simulink model "MdXX_RspOutComm"  (R2022b)
settings: Solver=FixedStepDiscrete  StartTime=0.0  StopTime=10.0  FixedStep=0.01  RelTol=1e-3
undefined symbols (not defined in the file or in its folder): KeSMSuRspStatHldTm_Val, MdRspLocal2, SrcReqTp1
libraries: simulink x64, RspLib x32
(part 2 of 5)

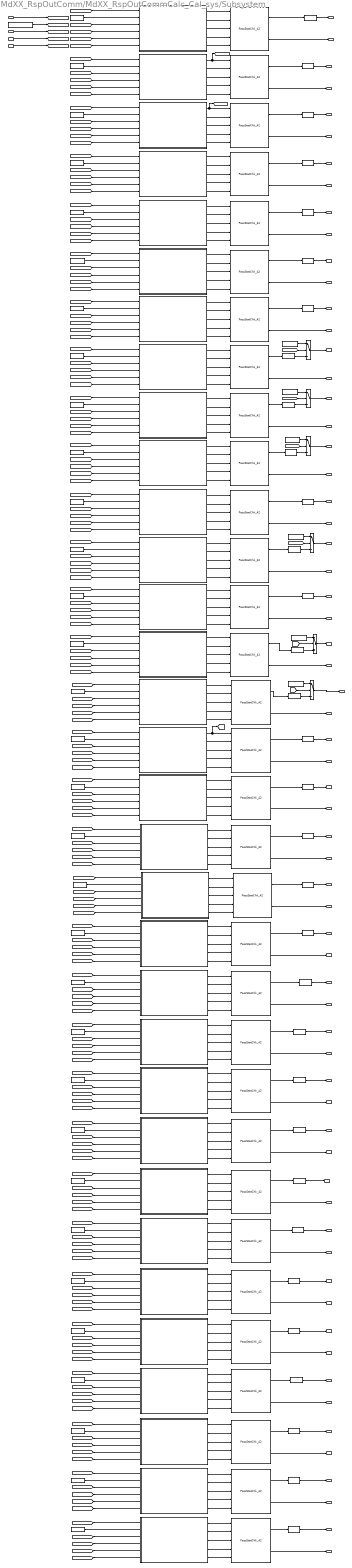
== system MdXX_RspOutComm/MdXX_RspOutCommCalc_Cal_sys/Subsystem ==
  MdXXIsTargetPosAlready_Val_read : Inport
  modestate32_Val_read : Inport  Port=2
  MdXX_QuitArray_Val_read : Inport  Port=3
  MdXX_SrcReqTpArray_Val_read : Inport  Port=4
  Constant{,32..37} (7 alike) : Constant  Value=0  OutDataTypeStr=uint8
  Constant1 : Constant  OutDataTypeStr=uint8
  Constant10 : Constant  Value=10  OutDataTypeStr=uint8
  Constant11 : Constant  Value=11  OutDataTypeStr=uint8
  Constant12 : Constant  Value=12  OutDataTypeStr=uint8
  Constant13 : Constant  Value=13  OutDataTypeStr=uint8
  Constant14 : Constant  Value=14  OutDataTypeStr=uint8
  Constant15 : Constant  Value=15  OutDataTypeStr=uint8
  Constant16 : Constant  Value=16  OutDataTypeStr=uint8
  Constant17 : Constant  Value=17  OutDataTypeStr=uint8
  Constant18 : Constant  Value=18  OutDataTypeStr=uint8
  Constant19 : Constant  Value=19  OutDataTypeStr=uint8
  Constant2 : Constant  Value=2  OutDataTypeStr=uint8
  Constant20 : Constant  Value=20  OutDataTypeStr=uint8
  Constant21 : Constant  Value=21  OutDataTypeStr=uint8
  Constant22 : Constant  Value=22  OutDataTypeStr=uint8
  Constant23 : Constant  Value=23  OutDataTypeStr=uint8
  Constant24 : Constant  Value=24  OutDataTypeStr=uint8
  Constant25 : Constant  Value=25  OutDataTypeStr=uint8
  Constant26 : Constant  Value=26  OutDataTypeStr=uint8
  Constant27 : Constant  Value=27  OutDataTypeStr=uint8
  Constant28 : Constant  Value=28  OutDataTypeStr=uint8
  Constant29 : Constant  Value=29  OutDataTypeStr=uint8
  Constant3 : Constant  Value=3  OutDataTypeStr=uint8
  Constant30 : Constant  Value=30  OutDataTypeStr=uint8
  Constant31 : Constant  Value=31  OutDataTypeStr=uint8
  Constant4 : Constant  Value=4  OutDataTypeStr=uint8
  Constant5 : Constant  Value=5  OutDataTypeStr=uint8
  Constant6 : Constant  Value=6  OutDataTypeStr=uint8
  Constant7 : Constant  Value=7  OutDataTypeStr=uint8
  Constant8 : Constant  Value=8  OutDataTypeStr=uint8
  Constant9 : Constant  Value=9  OutDataTypeStr=uint8
  Data Type Conversion{1..32} (32 alike) : DataTypeConversion  OutDataTypeStr=uint8  SaturateOnIntegerOverflow=off  RndMeth=Floor
  MdRsp{1..32} (32 alike) : RspLib/PassStatChk_42  SystemSampleTime=-1  VariantActivationTime=update diagram  Latency=0  AutoFrameSizeCalculation=off
  MdRspOutDataSelc1 : Subsystem
  MdRspOutDataSelc10 : Subsystem
  MdRspOutDataSelc11 : Subsystem
  MdRspOutDataSelc12 : Subsystem
  MdRspOutDataSelc13 : Subsystem
  MdRspOutDataSelc14 : Subsystem
  MdRspOutDataSelc15 : Subsystem
  MdRspOutDataSelc16 : Subsystem
  MdRspOutDataSelc17 : Subsystem
  MdRspOutDataSelc18 : Subsystem
  MdRspOutDataSelc19 : Subsystem
  MdRspOutDataSelc2 : Subsystem
  MdRspOutDataSelc20 : Subsystem
  MdRspOutDataSelc21 : Subsystem
  MdRspOutDataSelc22 : Subsystem
  MdRspOutDataSelc23 : Subsystem
  MdRspOutDataSelc24 : Subsystem
  MdRspOutDataSelc25 : Subsystem
  MdRspOutDataSelc26 : Subsystem
  MdRspOutDataSelc27 : Subsystem
  MdRspOutDataSelc28 : Subsystem
  MdRspOutDataSelc29 : Subsystem
  MdRspOutDataSelc3 : Subsystem
  MdRspOutDataSelc30 : Subsystem
  MdRspOutDataSelc31 : Subsystem
  MdRspOutDataSelc32 : Subsystem
  MdRspOutDataSelc4 : Subsystem
  MdRspOutDataSelc5 : Subsystem
  MdRspOutDataSelc6 : Subsystem
  MdRspOutDataSelc7 : Subsystem
  MdRspOutDataSelc8 : Subsystem
  MdRspOutDataSelc9 : Subsystem
  PA_KeSMSuRspStatHldTm_Val : Constant  Value=KeSMSuRspStatHldTm_Val
  Switch{,1..5} (6 alike) : Switch  Criteria=u2 > Threshold  SaturateOnIntegerOverflow=off  InputSameDT=off
  MdXX_RspOutComm_Md1_Rsp_write : Outport  VectorParamsAs1DForOutWhenUnconnected=off
      settings: EnsureOutportIsVirtual=on
  MdXX_RspOutComm_Md10_Rsp_write : Outport  Port=2  VectorParamsAs1DForOutWhenUnconnected=off
      settings: EnsureOutportIsVirtual=on
  MdXX_RspOutComm_Md11_Rsp_write : Outport  Port=3  VectorParamsAs1DForOutWhenUnconnected=off
      settings: EnsureOutportIsVirtual=on
  MdXX_RspOutComm_Md12_Rsp_write : Outport  Port=4  VectorParamsAs1DForOutWhenUnconnected=off
      settings: EnsureOutportIsVirtual=on
  MdXX_RspOutComm_Md13_Rsp_write : Outport  Port=5  VectorParamsAs1DForOutWhenUnconnected=off
      settings: EnsureOutportIsVirtual=on
  MdXX_RspOutComm_Md14_Rsp_write : Outport  Port=6  VectorParamsAs1DForOutWhenUnconnected=off
      settings: EnsureOutportIsVirtual=on
  MdXX_RspOutComm_Md15_Rsp_write : Outport  Port=7  VectorParamsAs1DForOutWhenUnconnected=off
      settings: EnsureOutportIsVirtual=on
  MdXX_RspOutComm_Md16_Rsp_write : Outport  Port=8  VectorParamsAs1DForOutWhenUnconnected=off
      settings: EnsureOutportIsVirtual=on
  MdXX_RspOutComm_Md17_Rsp_write : Outport  Port=9  VectorParamsAs1DForOutWhenUnconnected=off
      settings: EnsureOutportIsVirtual=on
  MdXX_RspOutComm_Md18_Rsp_write : Outport  Port=10  VectorParamsAs1DForOutWhenUnconnected=off
      settings: EnsureOutportIsVirtual=on
  MdXX_RspOutComm_Md19_Rsp_write : Outport  Port=11  VectorParamsAs1DForOutWhenUnconnected=off
      settings: EnsureOutportIsVirtual=on
  MdXX_RspOutComm_Md2_Rsp_write : Outport  Port=12  VectorParamsAs1DForOutWhenUnconnected=off
      settings: EnsureOutportIsVirtual=on
  MdXX_RspOutComm_Md20_Rsp_write : Outport  Port=13  VectorParamsAs1DForOutWhenUnconnected=off
      settings: EnsureOutportIsVirtual=on
  MdXX_RspOutComm_Md21_Rsp_write : Outport  Port=14  VectorParamsAs1DForOutWhenUnconnected=off
      settings: EnsureOutportIsVirtual=on
  MdXX_RspOutComm_Md22_Rsp_write : Outport  Port=15  VectorParamsAs1DForOutWhenUnconnected=off
      settings: EnsureOutportIsVirtual=on
  MdXX_RspOutComm_Md23_Rsp_write : Outport  Port=16  VectorParamsAs1DForOutWhenUnconnected=off
      settings: EnsureOutportIsVirtual=on
  MdXX_RspOutComm_Md24_Rsp_write : Outport  Port=17  VectorParamsAs1DForOutWhenUnconnected=off
      settings: EnsureOutportIsVirtual=on
  MdXX_RspOutComm_Md25_Rsp_write : Outport  Port=18  VectorParamsAs1DForOutWhenUnconnected=off
      settings: EnsureOutportIsVirtual=on
  MdXX_RspOutComm_Md26_Rsp_write : Outport  Port=19  VectorParamsAs1DForOutWhenUnconnected=off
      settings: EnsureOutportIsVirtual=on
  MdXX_RspOutComm_Md27_Rsp_write : Outport  Port=20  VectorParamsAs1DForOutWhenUnconnected=off
      settings: EnsureOutportIsVirtual=on
  MdXX_RspOutComm_Md28_Rsp_write : Outport  Port=21  VectorParamsAs1DForOutWhenUnconnected=off
      settings: EnsureOutportIsVirtual=on
  MdXX_RspOutComm_Md29_Rsp_write : Outport  Port=22  VectorParamsAs1DForOutWhenUnconnected=off
      settings: EnsureOutportIsVirtual=on
  MdXX_RspOutComm_Md3_Rsp_write : Outport  Port=23  VectorParamsAs1DForOutWhenUnconnected=off
      settings: EnsureOutportIsVirtual=on
  MdXX_RspOutComm_Md30_Rsp_write : Outport  Port=24  VectorParamsAs1DForOutWhenUnconnected=off
      settings: EnsureOutportIsVirtual=on
  MdXX_RspOutComm_Md31_Rsp_write : Outport  Port=25  VectorParamsAs1DForOutWhenUnconnected=off
      settings: EnsureOutportIsVirtual=on
  MdXX_RspOutComm_Md32_Rsp_write : Outport  Port=26  VectorParamsAs1DForOutWhenUnconnected=off
      settings: EnsureOutportIsVirtual=on
  MdXX_RspOutComm_Md4_Rsp_write : Outport  Port=27  VectorParamsAs1DForOutWhenUnconnected=off
      settings: EnsureOutportIsVirtual=on
  MdXX_RspOutComm_Md5_Rsp_write : Outport  Port=28  VectorParamsAs1DForOutWhenUnconnected=off
      settings: EnsureOutportIsVirtual=on
  MdXX_RspOutComm_Md6_Rsp_write : Outport  Port=29  VectorParamsAs1DForOutWhenUnconnected=off
      settings: EnsureOutportIsVirtual=on
  MdXX_RspOutComm_Md7_Rsp_write : Outport  Port=30  VectorParamsAs1DForOutWhenUnconnected=off
      settings: EnsureOutportIsVirtual=on
  MdXX_RspOutComm_Md8_Rsp_write : Outport  Port=31  VectorParamsAs1DForOutWhenUnconnected=off
      settings: EnsureOutportIsVirtual=on
  MdXX_RspOutComm_Md9_Rsp_write : Outport  Port=32  VectorParamsAs1DForOutWhenUnconnected=off
      settings: EnsureOutportIsVirtual=on
  MdXX_SrcReqTpOutComm_Md1_SrcTp_write : Outport  Port=33  VectorParamsAs1DForOutWhenUnconnected=off
      settings: EnsureOutportIsVirtual=on
  MdXX_SrcReqTpOutComm_Md10_SrcTp_write : Outport  Port=34  VectorParamsAs1DForOutWhenUnconnected=off
      settings: EnsureOutportIsVirtual=on
  MdXX_SrcReqTpOutComm_Md11_SrcTp_write : Outport  Port=35  VectorParamsAs1DForOutWhenUnconnected=off
      settings: EnsureOutportIsVirtual=on
  MdXX_SrcReqTpOutComm_Md12_SrcTp_write : Outport  Port=36  VectorParamsAs1DForOutWhenUnconnected=off
      settings: EnsureOutportIsVirtual=on
  MdXX_SrcReqTpOutComm_Md13_SrcTp_write : Outport  Port=37  VectorParamsAs1DForOutWhenUnconnected=off
      settings: EnsureOutportIsVirtual=on
  MdXX_SrcReqTpOutComm_Md14_SrcTp_write : Outport  Port=38  VectorParamsAs1DForOutWhenUnconnected=off
      settings: EnsureOutportIsVirtual=on
  MdXX_SrcReqTpOutComm_Md15_SrcTp_write : Outport  Port=39  VectorParamsAs1DForOutWhenUnconnected=off
      settings: EnsureOutportIsVirtual=on
  MdXX_SrcReqTpOutComm_Md16_SrcTp_write : Outport  Port=40  VectorParamsAs1DForOutWhenUnconnected=off
      settings: EnsureOutportIsVirtual=on
  MdXX_SrcReqTpOutComm_Md17_SrcTp_write : Outport  Port=41  VectorParamsAs1DForOutWhenUnconnected=off
      settings: EnsureOutportIsVirtual=on
  MdXX_SrcReqTpOutComm_Md18_SrcTp_write : Outport  Port=42  VectorParamsAs1DForOutWhenUnconnected=off
      settings: EnsureOutportIsVirtual=on
  MdXX_SrcReqTpOutComm_Md19_SrcTp_write : Outport  Port=43  VectorParamsAs1DForOutWhenUnconnected=off
      settings: EnsureOutportIsVirtual=on
  MdXX_SrcReqTpOutComm_Md2_SrcTp_write : Outport  Port=44  VectorParamsAs1DForOutWhenUnconnected=off
      settings: EnsureOutportIsVirtual=on
  MdXX_SrcReqTpOutComm_Md20_SrcTp_write : Outport  Port=45  VectorParamsAs1DForOutWhenUnconnected=off
      settings: EnsureOutportIsVirtual=on
  MdXX_SrcReqTpOutComm_Md21_SrcTp_write : Outport  Port=46  VectorParamsAs1DForOutWhenUnconnected=off
      settings: EnsureOutportIsVirtual=on
  MdXX_SrcReqTpOutComm_Md22_SrcTp_write : Outport  Port=47  VectorParamsAs1DForOutWhenUnconnected=off
      settings: EnsureOutportIsVirtual=on
  MdXX_SrcReqTpOutComm_Md23_SrcTp_write : Outport  Port=48  VectorParamsAs1DForOutWhenUnconnected=off
      settings: EnsureOutportIsVirtual=on
  MdXX_SrcReqTpOutComm_Md24_SrcTp_write : Outport  Port=49  VectorParamsAs1DForOutWhenUnconnected=off
      settings: EnsureOutportIsVirtual=on
  MdXX_SrcReqTpOutComm_Md25_SrcTp_write : Outport  Port=50  VectorParamsAs1DForOutWhenUnconnected=off
      settings: EnsureOutportIsVirtual=on
  MdXX_SrcReqTpOutComm_Md26_SrcTp_write : Outport  Port=51  VectorParamsAs1DForOutWhenUnconnected=off
      settings: EnsureOutportIsVirtual=on
  MdXX_SrcReqTpOutComm_Md27_SrcTp_write : Outport  Port=52  VectorParamsAs1DForOutWhenUnconnected=off
      settings: EnsureOutportIsVirtual=on
  MdXX_SrcReqTpOutComm_Md28_SrcTp_write : Outport  Port=53  VectorParamsAs1DForOutWhenUnconnected=off
      settings: EnsureOutportIsVirtual=on
  MdXX_SrcReqTpOutComm_Md29_SrcTp_write : Outport  Port=54  VectorParamsAs1DForOutWhenUnconnected=off
      settings: EnsureOutportIsVirtual=on
  MdXX_SrcReqTpOutComm_Md3_SrcTp_write : Outport  Port=55  VectorParamsAs1DForOutWhenUnconnected=off
      settings: EnsureOutportIsVirtual=on
  MdXX_SrcReqTpOutComm_Md30_SrcTp_write : Outport  Port=56  VectorParamsAs1DForOutWhenUnconnected=off
      settings: EnsureOutportIsVirtual=on
  MdXX_SrcReqTpOutComm_Md31_SrcTp_write : Outport  Port=57  VectorParamsAs1DForOutWhenUnconnected=off
      settings: EnsureOutportIsVirtual=on
  MdXX_SrcReqTpOutComm_Md32_SrcTp_write : Outport  Port=58  VectorParamsAs1DForOutWhenUnconnected=off
      settings: EnsureOutportIsVirtual=on
  MdXX_SrcReqTpOutComm_Md4_SrcTp_write : Outport  Port=59  VectorParamsAs1DForOutWhenUnconnected=off
      settings: EnsureOutportIsVirtual=on
  MdXX_SrcReqTpOutComm_Md5_SrcTp_write : Outport  Port=60  VectorParamsAs1DForOutWhenUnconnected=off
      settings: EnsureOutportIsVirtual=on
  MdXX_SrcReqTpOutComm_Md6_SrcTp_write : Outport  Port=61  VectorParamsAs1DForOutWhenUnconnected=off
      settings: EnsureOutportIsVirtual=on
  MdXX_SrcReqTpOutComm_Md7_SrcTp_write : Outport  Port=62  VectorParamsAs1DForOutWhenUnconnected=off
      settings: EnsureOutportIsVirtual=on
  MdXX_SrcReqTpOutComm_Md8_SrcTp_write : Outport  Port=63  VectorParamsAs1DForOutWhenUnconnected=off
      settings: EnsureOutportIsVirtual=on
  MdXX_SrcReqTpOutComm_Md9_SrcTp_write : Outport  Port=64  VectorParamsAs1DForOutWhenUnconnected=off
      settings: EnsureOutportIsVirtual=on
  wires:
  MdRsp16/1 -> Data Type Conversion16/1
  MdRsp10/1 -> Data Type Conversion10/1
  MdRsp13/1 -> Data Type Conversion13/1
  MdRsp18/1 -> Data Type Conversion18/1
  MdRsp12/1 -> Data Type Conversion12/1
  MdRsp17/1 -> Data Type Conversion17/1
  MdRsp19/1 -> Data Type Conversion19/1
  MdRsp11/1 -> Data Type Conversion11/1
  MdRsp20/1 -> Data Type Conversion20/1
  MdRsp1/1 -> Data Type Conversion1/1
  MdRsp2/1 -> Data Type Conversion2/1
  MdRsp3/1 -> Data Type Conversion4/1
  MdRsp4/1 -> Data Type Conversion3/1
  MdRsp5/1 -> Data Type Conversion5/1
  MdRsp6/1 -> Data Type Conversion6/1
  MdRsp7/1 -> Data Type Conversion7/1
  MdRsp8/1 -> Data Type Conversion8/1
  MdRsp9/1 -> Data Type Conversion9/1
  MdRsp1/2 -> MdXX_SrcReqTpOutComm_Md1_SrcTp_write/1
  MdRsp4/2 -> MdXX_SrcReqTpOutComm_Md4_SrcTp_write/1
  MdRsp5/2 -> MdXX_SrcReqTpOutComm_Md5_SrcTp_write/1
  MdRsp6/2 -> MdXX_SrcReqTpOutComm_Md6_SrcTp_write/1
  MdRsp7/2 -> MdXX_SrcReqTpOutComm_Md7_SrcTp_write/1
  MdRsp8/2 -> MdXX_SrcReqTpOutComm_Md8_SrcTp_write/1
  MdRsp9/2 -> MdXX_SrcReqTpOutComm_Md9_SrcTp_write/1
  MdRsp10/2 -> MdXX_SrcReqTpOutComm_Md10_SrcTp_write/1
  MdRsp11/2 -> MdXX_SrcReqTpOutComm_Md11_SrcTp_write/1
  MdRsp12/2 -> MdXX_SrcReqTpOutComm_Md12_SrcTp_write/1
  MdRsp13/2 -> MdXX_SrcReqTpOutComm_Md13_SrcTp_write/1
  MdRsp14/2 -> MdXX_SrcReqTpOutComm_Md14_SrcTp_write/1
  MdRsp15/2 -> MdXX_SrcReqTpOutComm_Md15_SrcTp_write/1
  MdRsp16/2 -> MdXX_SrcReqTpOutComm_Md16_SrcTp_write/1
  MdRsp17/2 -> MdXX_SrcReqTpOutComm_Md17_SrcTp_write/1
  MdRsp18/2 -> MdXX_SrcReqTpOutComm_Md18_SrcTp_write/1
  MdRsp19/2 -> MdXX_SrcReqTpOutComm_Md19_SrcTp_write/1
  MdRsp20/2 -> MdXX_SrcReqTpOutComm_Md20_SrcTp_write/1
  MdRsp2/2 -> MdXX_SrcReqTpOutComm_Md2_SrcTp_write/1
  MdRsp3/2 -> MdXX_SrcReqTpOutComm_Md3_SrcTp_write/1
  Data Type Conversion3/1 -> MdXX_RspOutComm_Md4_Rsp_write/1
  Data Type Conversion4/1 -> MdXX_RspOutComm_Md3_Rsp_write/1
  Data Type Conversion2/1 -> MdXX_RspOutComm_Md2_Rsp_write/1
  Data Type Conversion1/1 -> MdXX_RspOutComm_Md1_Rsp_write/1
  Data Type Conversion5/1 -> MdXX_RspOutComm_Md5_Rsp_write/1
  Data Type Conversion6/1 -> MdXX_RspOutComm_Md6_Rsp_write/1
  Data Type Conversion7/1 -> MdXX_RspOutComm_Md7_Rsp_write/1
  Data Type Conversion11/1 -> MdXX_RspOutComm_Md11_Rsp_write/1
  Data Type Conversion13/1 -> MdXX_RspOutComm_Md13_Rsp_write/1
  Switch5/1 -> MdXX_RspOutComm_Md15_Rsp_write/1
  Data Type Conversion16/1 -> MdXX_RspOutComm_Md16_Rsp_write/1
  Data Type Conversion17/1 -> MdXX_RspOutComm_Md17_Rsp_write/1
  Data Type Conversion18/1 -> MdXX_RspOutComm_Md18_Rsp_write/1
  Data Type Conversion19/1 -> MdXX_RspOutComm_Md19_Rsp_write/1
  Data Type Conversion20/1 -> MdXX_RspOutComm_Md20_Rsp_write/1
  MdRsp32/2 -> MdXX_SrcReqTpOutComm_Md32_SrcTp_write/1
  MdRsp31/2 -> MdXX_SrcReqTpOutComm_Md31_SrcTp_write/1
  MdRsp30/2 -> MdXX_SrcReqTpOutComm_Md30_SrcTp_write/1
  MdRsp29/2 -> MdXX_SrcReqTpOutComm_Md29_SrcTp_write/1
  MdRsp28/2 -> MdXX_SrcReqTpOutComm_Md28_SrcTp_write/1
  MdRsp27/2 -> MdXX_SrcReqTpOutComm_Md27_SrcTp_write/1
  MdRsp26/2 -> MdXX_SrcReqTpOutComm_Md26_SrcTp_write/1
  MdRsp25/2 -> MdXX_SrcReqTpOutComm_Md25_SrcTp_write/1
  MdRsp24/2 -> MdXX_SrcReqTpOutComm_Md24_SrcTp_write/1
  MdRsp23/2 -> MdXX_SrcReqTpOutComm_Md23_SrcTp_write/1
  MdRsp22/2 -> MdXX_SrcReqTpOutComm_Md22_SrcTp_write/1
  MdRsp21/2 -> MdXX_SrcReqTpOutComm_Md21_SrcTp_write/1
  MdRspOutDataSelc1/1(MdEn) -> MdRsp1/1
  MdRspOutDataSelc1/2(HldTm) -> MdRsp1/2
  MdRspOutDataSelc1/3(Rsp) -> MdRsp1/3
  MdRspOutDataSelc1/4(IsTrgtPos) -> MdRsp1/4
  MdRspOutDataSelc1/5(SrcReqTp) -> MdRsp1/5
  MdRspOutDataSelc2/5(SrcReqTp) -> MdRsp2/5
  MdRspOutDataSelc2/4(IsTrgtPos) -> MdRsp2/4
  MdRspOutDataSelc2/3(Rsp) -> MdRsp2/3
  MdRspOutDataSelc3/3(Rsp) -> MdRsp3/3
  MdRspOutDataSelc3/4(IsTrgtPos) -> MdRsp3/4
  MdRspOutDataSelc3/5(SrcReqTp) -> MdRsp3/5
  MdRspOutDataSelc4/5(SrcReqTp) -> MdRsp4/5
  MdRspOutDataSelc4/4(IsTrgtPos) -> MdRsp4/4
  MdRspOutDataSelc4/3(Rsp) -> MdRsp4/3
  MdRspOutDataSelc5/3(Rsp) -> MdRsp5/3
  MdRspOutDataSelc5/4(IsTrgtPos) -> MdRsp5/4
  MdRspOutDataSelc5/5(SrcReqTp) -> MdRsp5/5
  MdRspOutDataSelc6/5(SrcReqTp) -> MdRsp6/5
  MdRspOutDataSelc6/4(IsTrgtPos) -> MdRsp6/4
  MdRspOutDataSelc6/3(Rsp) -> MdRsp6/3
  MdRspOutDataSelc7/3(Rsp) -> MdRsp7/3
  MdRspOutDataSelc7/4(IsTrgtPos) -> MdRsp7/4
  MdRspOutDataSelc7/5(SrcReqTp) -> MdRsp7/5
  MdRspOutDataSelc8/5(SrcReqTp) -> MdRsp8/5
  MdRspOutDataSelc8/4(IsTrgtPos) -> MdRsp8/4
  MdRspOutDataSelc8/3(Rsp) -> MdRsp8/3
  MdRspOutDataSelc9/3(Rsp) -> MdRsp9/3
  MdRspOutDataSelc9/4(IsTrgtPos) -> MdRsp9/4
  MdRspOutDataSelc9/5(SrcReqTp) -> MdRsp9/5
  MdRspOutDataSelc10/5(SrcReqTp) -> MdRsp10/5
  MdRspOutDataSelc10/4(IsTrgtPos) -> MdRsp10/4
  MdRspOutDataSelc10/3(Rsp) -> MdRsp10/3
  MdRspOutDataSelc11/3(Rsp) -> MdRsp11/3
  MdRspOutDataSelc11/4(IsTrgtPos) -> MdRsp11/4
  MdRspOutDataSelc11/5(SrcReqTp) -> MdRsp11/5
  MdRspOutDataSelc12/5(SrcReqTp) -> MdRsp12/5
  MdRspOutDataSelc12/4(IsTrgtPos) -> MdRsp12/4
  MdRspOutDataSelc12/3(Rsp) -> MdRsp12/3
  MdRspOutDataSelc13/3(Rsp) -> MdRsp13/3
  MdRspOutDataSelc13/4(IsTrgtPos) -> MdRsp13/4
  MdRspOutDataSelc13/5(SrcReqTp) -> MdRsp13/5
  modestate32_Val_read/1 -> [modestate32]
  Constant/1 -> MdRspOutDataSelc1/2(Index)
  [modestate32] -> MdRspOutDataSelc1/1(modestate32_Val_read)
  PA_KeSMSuRspStatHldTm_Val/1 -> [KeSMSuRspStatHldTm_Val]
  MdXX_QuitArray_Val_read/1 -> [MdXX_QuitArray]
  MdXXIsTargetPosAlready_Val_read/1 -> [MdXXIsTargetPosAlready]
  MdXX_SrcReqTpArray_Val_read/1 -> [MdXX_SrcReqTpArray]
  [KeSMSuRspStatHldTm_Val] -> MdRspOutDataSelc1/3(KeSMSuRspStatHldTm_Val)
  [MdXX_QuitArray] -> MdRspOutDataSelc1/4(QuitArray)
  [MdXXIsTargetPosAlready] -> MdRspOutDataSelc1/5(IsTargetPos32Bit_Val_read)
  [MdXX_SrcReqTpArray] -> MdRspOutDataSelc1/6(SrcReqTpArray)
  [modestate32] -> MdRspOutDataSelc2/1(modestate32_Val_read)
  [MdXX_QuitArray] -> MdRspOutDataSelc2/4(QuitArray)
  [MdXXIsTargetPosAlready] -> MdRspOutDataSelc2/5(IsTargetPos32Bit_Val_read)
  Constant1/1 -> MdRspOutDataSelc2/2(Index)
  [MdXX_SrcReqTpArray] -> MdRspOutDataSelc2/6(SrcReqTpArray)
  [KeSMSuRspStatHldTm_Val] -> MdRspOutDataSelc2/3(KeSMSuRspStatHldTm_Val)
  [modestate32] -> MdRspOutDataSelc3/1(modestate32_Val_read)
  [MdXX_QuitArray] -> MdRspOutDataSelc3/4(QuitArray)
  [MdXXIsTargetPosAlready] -> MdRspOutDataSelc3/5(IsTargetPos32Bit_Val_read)
  Constant2/1 -> MdRspOutDataSelc3/2(Index)
  [MdXX_SrcReqTpArray] -> MdRspOutDataSelc3/6(SrcReqTpArray)
  [KeSMSuRspStatHldTm_Val] -> MdRspOutDataSelc3/3(KeSMSuRspStatHldTm_Val)
  [modestate32] -> MdRspOutDataSelc4/1(modestate32_Val_read)
  [MdXX_QuitArray] -> MdRspOutDataSelc4/4(QuitArray)
  [MdXXIsTargetPosAlready] -> MdRspOutDataSelc4/5(IsTargetPos32Bit_Val_read)
  Constant3/1 -> MdRspOutDataSelc4/2(Index)
  [MdXX_SrcReqTpArray] -> MdRspOutDataSelc4/6(SrcReqTpArray)
  [KeSMSuRspStatHldTm_Val] -> MdRspOutDataSelc4/3(KeSMSuRspStatHldTm_Val)
  [modestate32] -> MdRspOutDataSelc5/1(modestate32_Val_read)
  [MdXX_QuitArray] -> MdRspOutDataSelc5/4(QuitArray)
  [MdXXIsTargetPosAlready] -> MdRspOutDataSelc5/5(IsTargetPos32Bit_Val_read)
  Constant4/1 -> MdRspOutDataSelc5/2(Index)
  [MdXX_SrcReqTpArray] -> MdRspOutDataSelc5/6(SrcReqTpArray)
  [KeSMSuRspStatHldTm_Val] -> MdRspOutDataSelc5/3(KeSMSuRspStatHldTm_Val)
  [modestate32] -> MdRspOutDataSelc6/1(modestate32_Val_read)
  [MdXX_QuitArray] -> MdRspOutDataSelc6/4(QuitArray)
  [MdXXIsTargetPosAlready] -> MdRspOutDataSelc6/5(IsTargetPos32Bit_Val_read)
  Constant5/1 -> MdRspOutDataSelc6/2(Index)
  [MdXX_SrcReqTpArray] -> MdRspOutDataSelc6/6(SrcReqTpArray)
  [KeSMSuRspStatHldTm_Val] -> MdRspOutDataSelc6/3(KeSMSuRspStatHldTm_Val)
  [modestate32] -> MdRspOutDataSelc7/1(modestate32_Val_read)
  [MdXX_QuitArray] -> MdRspOutDataSelc7/4(QuitArray)
  [MdXXIsTargetPosAlready] -> MdRspOutDataSelc7/5(IsTargetPos32Bit_Val_read)
  Constant6/1 -> MdRspOutDataSelc7/2(Index)
  [MdXX_SrcReqTpArray] -> MdRspOutDataSelc7/6(SrcReqTpArray)
  [KeSMSuRspStatHldTm_Val] -> MdRspOutDataSelc7/3(KeSMSuRspStatHldTm_Val)
  [modestate32] -> MdRspOutDataSelc8/1(modestate32_Val_read)
  [MdXX_QuitArray] -> MdRspOutDataSelc8/4(QuitArray)
  [MdXXIsTargetPosAlready] -> MdRspOutDataSelc8/5(IsTargetPos32Bit_Val_read)
  Constant7/1 -> MdRspOutDataSelc8/2(Index)
  [MdXX_SrcReqTpArray] -> MdRspOutDataSelc8/6(SrcReqTpArray)
  [KeSMSuRspStatHldTm_Val] -> MdRspOutDataSelc8/3(KeSMSuRspStatHldTm_Val)
  [modestate32] -> MdRspOutDataSelc9/1(modestate32_Val_read)
  [MdXX_QuitArray] -> MdRspOutDataSelc9/4(QuitArray)
  [MdXXIsTargetPosAlready] -> MdRspOutDataSelc9/5(IsTargetPos32Bit_Val_read)
  Constant8/1 -> MdRspOutDataSelc9/2(Index)
  [MdXX_SrcReqTpArray] -> MdRspOutDataSelc9/6(SrcReqTpArray)
  [KeSMSuRspStatHldTm_Val] -> MdRspOutDataSelc9/3(KeSMSuRspStatHldTm_Val)
  [modestate32] -> MdRspOutDataSelc10/1(modestate32_Val_read)
  [MdXX_QuitArray] -> MdRspOutDataSelc10/4(QuitArray)
  [MdXXIsTargetPosAlready] -> MdRspOutDataSelc10/5(IsTargetPos32Bit_Val_read)
  Constant9/1 -> MdRspOutDataSelc10/2(Index)
  [MdXX_SrcReqTpArray] -> MdRspOutDataSelc10/6(SrcReqTpArray)
  [KeSMSuRspStatHldTm_Val] -> MdRspOutDataSelc10/3(KeSMSuRspStatHldTm_Val)
  [modestate32] -> MdRspOutDataSelc11/1(modestate32_Val_read)
  [MdXX_QuitArray] -> MdRspOutDataSelc11/4(QuitArray)
  [MdXXIsTargetPosAlready] -> MdRspOutDataSelc11/5(IsTargetPos32Bit_Val_read)
  Constant10/1 -> MdRspOutDataSelc11/2(Index)
  [MdXX_SrcReqTpArray] -> MdRspOutDataSelc11/6(SrcReqTpArray)
  [KeSMSuRspStatHldTm_Val] -> MdRspOutDataSelc11/3(KeSMSuRspStatHldTm_Val)
  [modestate32] -> MdRspOutDataSelc12/1(modestate32_Val_read)
  [MdXX_QuitArray] -> MdRspOutDataSelc12/4(QuitArray)
  [MdXXIsTargetPosAlready] -> MdRspOutDataSelc12/5(IsTargetPos32Bit_Val_read)
  Constant11/1 -> MdRspOutDataSelc12/2(Index)
  [MdXX_SrcReqTpArray] -> MdRspOutDataSelc12/6(SrcReqTpArray)
  [KeSMSuRspStatHldTm_Val] -> MdRspOutDataSelc12/3(KeSMSuRspStatHldTm_Val)
  [modestate32] -> MdRspOutDataSelc13/1(modestate32_Val_read)
  [MdXX_QuitArray] -> MdRspOutDataSelc13/4(QuitArray)
  [MdXXIsTargetPosAlready] -> MdRspOutDataSelc13/5(IsTargetPos32Bit_Val_read)
  Constant12/1 -> MdRspOutDataSelc13/2(Index)
  [MdXX_SrcReqTpArray] -> MdRspOutDataSelc13/6(SrcReqTpArray)
  [KeSMSuRspStatHldTm_Val] -> MdRspOutDataSelc13/3(KeSMSuRspStatHldTm_Val)
  MdRspOutDataSelc13/1(MdEn) -> MdRsp13/1
  MdRspOutDataSelc13/2(HldTm) -> MdRsp13/2
  MdRspOutDataSelc12/1(MdEn) -> MdRsp12/1
  MdRspOutDataSelc12/2(HldTm) -> MdRsp12/2
  MdRspOutDataSelc11/1(MdEn) -> MdRsp11/1
  MdRspOutDataSelc11/2(HldTm) -> MdRsp11/2
  MdRspOutDataSelc10/1(MdEn) -> MdRsp10/1
  MdRspOutDataSelc10/2(HldTm) -> MdRsp10/2
  MdRspOutDataSelc9/1(MdEn) -> MdRsp9/1
  MdRspOutDataSelc9/2(HldTm) -> MdRsp9/2
  MdRspOutDataSelc8/1(MdEn) -> MdRsp8/1
  MdRspOutDataSelc8/2(HldTm) -> MdRsp8/2
  MdRspOutDataSelc7/1(MdEn) -> MdRsp7/1
  MdRspOutDataSelc7/2(HldTm) -> MdRsp7/2
  MdRspOutDataSelc6/1(MdEn) -> MdRsp6/1
  MdRspOutDataSelc6/2(HldTm) -> MdRsp6/2
  MdRspOutDataSelc5/1(MdEn) -> MdRsp5/1
  MdRspOutDataSelc5/2(HldTm) -> MdRsp5/2
  MdRspOutDataSelc4/1(MdEn) -> MdRsp4/1
  MdRspOutDataSelc4/2(HldTm) -> MdRsp4/2
  MdRspOutDataSelc3/1(MdEn) -> [LugAllEn], MdRsp3/1
  MdRspOutDataSelc3/2(HldTm) -> MdRsp3/2
  MdRspOutDataSelc2/1(MdEn) -> [VIPAllEn], MdRsp2/1
  MdRspOutDataSelc2/2(HldTm) -> MdRsp2/2
  MdRspOutDataSelc14/2(HldTm) -> MdRsp14/2
  MdRspOutDataSelc14/1(MdEn) -> MdRsp14/1
  [KeSMSuRspStatHldTm_Val] -> MdRspOutDataSelc14/3(KeSMSuRspStatHldTm_Val)
  [MdXX_SrcReqTpArray] -> MdRspOutDataSelc14/6(SrcReqTpArray)
  Constant13/1 -> MdRspOutDataSelc14/2(Index)
  [MdXXIsTargetPosAlready] -> MdRspOutDataSelc14/5(IsTargetPos32Bit_Val_read)
  [MdXX_QuitArray] -> MdRspOutDataSelc14/4(QuitArray)
  [modestate32] -> MdRspOutDataSelc14/1(modestate32_Val_read)
  MdRspOutDataSelc14/5(SrcReqTp) -> MdRsp14/5
  MdRspOutDataSelc14/4(IsTrgtPos) -> MdRsp14/4
  MdRspOutDataSelc14/3(Rsp) -> MdRsp14/3
  MdRspOutDataSelc15/3(Rsp) -> MdRsp15/3
  MdRspOutDataSelc15/4(IsTrgtPos) -> MdRsp15/4
  MdRspOutDataSelc15/5(SrcReqTp) -> MdRsp15/5
  [modestate32] -> MdRspOutDataSelc15/1(modestate32_Val_read)
  [MdXX_QuitArray] -> MdRspOutDataSelc15/4(QuitArray)
  [MdXXIsTargetPosAlready] -> MdRspOutDataSelc15/5(IsTargetPos32Bit_Val_read)
  Constant14/1 -> MdRspOutDataSelc15/2(Index)
  [MdXX_SrcReqTpArray] -> MdRspOutDataSelc15/6(SrcReqTpArray)
  [KeSMSuRspStatHldTm_Val] -> MdRspOutDataSelc15/3(KeSMSuRspStatHldTm_Val)
  MdRspOutDataSelc15/1(MdEn) -> MdRsp15/1
  MdRspOutDataSelc15/2(HldTm) -> MdRsp15/2
  MdRspOutDataSelc16/2(HldTm) -> MdRsp16/2
  MdRspOutDataSelc16/1(MdEn) -> [bed], MdRsp16/1
  [KeSMSuRspStatHldTm_Val] -> MdRspOutDataSelc16/3(KeSMSuRspStatHldTm_Val)
  [MdXX_SrcReqTpArray] -> MdRspOutDataSelc16/6(SrcReqTpArray)
  Constant15/1 -> MdRspOutDataSelc16/2(Index)
  [MdXXIsTargetPosAlready] -> MdRspOutDataSelc16/5(IsTargetPos32Bit_Val_read)
  [MdXX_QuitArray] -> MdRspOutDataSelc16/4(QuitArray)
  [modestate32] -> MdRspOutDataSelc16/1(modestate32_Val_read)
  MdRspOutDataSelc16/5(SrcReqTp) -> MdRsp16/5
  MdRspOutDataSelc16/4(IsTrgtPos) -> MdRsp16/4
  MdRspOutDataSelc16/3(Rsp) -> MdRsp16/3
  MdRspOutDataSelc17/3(Rsp) -> MdRsp17/3
  MdRspOutDataSelc17/4(IsTrgtPos) -> MdRsp17/4
  MdRspOutDataSelc17/5(SrcReqTp) -> MdRsp17/5
  [modestate32] -> MdRspOutDataSelc17/1(modestate32_Val_read)
  [MdXX_QuitArray] -> MdRspOutDataSelc17/4(QuitArray)
  [MdXXIsTargetPosAlready] -> MdRspOutDataSelc17/5(IsTargetPos32Bit_Val_read)
  Constant16/1 -> MdRspOutDataSelc17/2(Index)
  [MdXX_SrcReqTpArray] -> MdRspOutDataSelc17/6(SrcReqTpArray)
  [KeSMSuRspStatHldTm_Val] -> MdRspOutDataSelc17/3(KeSMSuRspStatHldTm_Val)
  MdRspOutDataSelc17/1(MdEn) -> MdRsp17/1
  MdRspOutDataSelc17/2(HldTm) -> MdRsp17/2
  MdRspOutDataSelc18/2(HldTm) -> MdRsp18/2
  MdRspOutDataSelc18/1(MdEn) -> MdRsp18/1
  [KeSMSuRspStatHldTm_Val] -> MdRspOutDataSelc18/3(KeSMSuRspStatHldTm_Val)
  [MdXX_SrcReqTpArray] -> MdRspOutDataSelc18/6(SrcReqTpArray)
  Constant17/1 -> MdRspOutDataSelc18/2(Index)
  [MdXXIsTargetPosAlready] -> MdRspOutDataSelc18/5(IsTargetPos32Bit_Val_read)
  [MdXX_QuitArray] -> MdRspOutDataSelc18/4(QuitArray)
  [modestate32] -> MdRspOutDataSelc18/1(modestate32_Val_read)
  MdRspOutDataSelc18/5(SrcReqTp) -> MdRsp18/5
  MdRspOutDataSelc18/4(IsTrgtPos) -> MdRsp18/4
  MdRspOutDataSelc18/3(Rsp) -> MdRsp18/3
  MdRspOutDataSelc19/3(Rsp) -> MdRsp19/3
  MdRspOutDataSelc19/4(IsTrgtPos) -> MdRsp19/4
  MdRspOutDataSelc19/5(SrcReqTp) -> MdRsp19/5
  [modestate32] -> MdRspOutDataSelc19/1(modestate32_Val_read)
  [MdXX_QuitArray] -> MdRspOutDataSelc19/4(QuitArray)
  [MdXXIsTargetPosAlready] -> MdRspOutDataSelc19/5(IsTargetPos32Bit_Val_read)
  Constant18/1 -> MdRspOutDataSelc19/2(Index)
  [MdXX_SrcReqTpArray] -> MdRspOutDataSelc19/6(SrcReqTpArray)
  [KeSMSuRspStatHldTm_Val] -> MdRspOutDataSelc19/3(KeSMSuRspStatHldTm_Val)
  MdRspOutDataSelc19/1(MdEn) -> MdRsp19/1
  MdRspOutDataSelc19/2(HldTm) -> MdRsp19/2
  MdRspOutDataSelc20/2(HldTm) -> MdRsp20/2
  MdRspOutDataSelc20/1(MdEn) -> MdRsp20/1
  [KeSMSuRspStatHldTm_Val] -> MdRspOutDataSelc20/3(KeSMSuRspStatHldTm_Val)
  [MdXX_SrcReqTpArray] -> MdRspOutDataSelc20/6(SrcReqTpArray)
  Constant19/1 -> MdRspOutDataSelc20/2(Index)
  [MdXXIsTargetPosAlready] -> MdRspOutDataSelc20/5(IsTargetPos32Bit_Val_read)
  [MdXX_QuitArray] -> MdRspOutDataSelc20/4(QuitArray)
  [modestate32] -> MdRspOutDataSelc20/1(modestate32_Val_read)
  MdRspOutDataSelc20/5(SrcReqTp) -> MdRsp20/5
  MdRspOutDataSelc20/4(IsTrgtPos) -> MdRsp20/4
  MdRspOutDataSelc20/3(Rsp) -> MdRsp20/3
  MdRspOutDataSelc21/3(Rsp) -> MdRsp21/3
  MdRspOutDataSelc21/4(IsTrgtPos) -> MdRsp21/4
  MdRspOutDataSelc21/5(SrcReqTp) -> MdRsp21/5
  [modestate32] -> MdRspOutDataSelc21/1(modestate32_Val_read)
  [MdXX_QuitArray] -> MdRspOutDataSelc21/4(QuitArray)
  [MdXXIsTargetPosAlready] -> MdRspOutDataSelc21/5(IsTargetPos32Bit_Val_read)
  Constant20/1 -> MdRspOutDataSelc21/2(Index)
  [MdXX_SrcReqTpArray] -> MdRspOutDataSelc21/6(SrcReqTpArray)
  [KeSMSuRspStatHldTm_Val] -> MdRspOutDataSelc21/3(KeSMSuRspStatHldTm_Val)
  MdRspOutDataSelc21/1(MdEn) -> MdRsp21/1
  MdRspOutDataSelc21/2(HldTm) -> MdRsp21/2
  MdRspOutDataSelc22/2(HldTm) -> MdRsp22/2
  MdRspOutDataSelc22/1(MdEn) -> MdRsp22/1
  [KeSMSuRspStatHldTm_Val] -> MdRspOutDataSelc22/3(KeSMSuRspStatHldTm_Val)
  [MdXX_SrcReqTpArray] -> MdRspOutDataSelc22/6(SrcReqTpArray)
  Constant21/1 -> MdRspOutDataSelc22/2(Index)
  [MdXXIsTargetPosAlready] -> MdRspOutDataSelc22/5(IsTargetPos32Bit_Val_read)
  [MdXX_QuitArray] -> MdRspOutDataSelc22/4(QuitArray)
  [modestate32] -> MdRspOutDataSelc22/1(modestate32_Val_read)
  MdRspOutDataSelc22/5(SrcReqTp) -> MdRsp22/5
  MdRspOutDataSelc22/4(IsTrgtPos) -> MdRsp22/4
  MdRspOutDataSelc22/3(Rsp) -> MdRsp22/3
  MdRspOutDataSelc23/3(Rsp) -> MdRsp23/3
  MdRspOutDataSelc23/4(IsTrgtPos) -> MdRsp23/4
  MdRspOutDataSelc23/5(SrcReqTp) -> MdRsp23/5
  [modestate32] -> MdRspOutDataSelc23/1(modestate32_Val_read)
  [MdXX_QuitArray] -> MdRspOutDataSelc23/4(QuitArray)
  [MdXXIsTargetPosAlready] -> MdRspOutDataSelc23/5(IsTargetPos32Bit_Val_read)
  Constant22/1 -> MdRspOutDataSelc23/2(Index)
  [MdXX_SrcReqTpArray] -> MdRspOutDataSelc23/6(SrcReqTpArray)
  [KeSMSuRspStatHldTm_Val] -> MdRspOutDataSelc23/3(KeSMSuRspStatHldTm_Val)
  MdRspOutDataSelc23/1(MdEn) -> MdRsp23/1
  MdRspOutDataSelc23/2(HldTm) -> MdRsp23/2
  MdRspOutDataSelc24/2(HldTm) -> MdRsp24/2
  MdRspOutDataSelc24/1(MdEn) -> MdRsp24/1
  [KeSMSuRspStatHldTm_Val] -> MdRspOutDataSelc24/3(KeSMSuRspStatHldTm_Val)
  [MdXX_SrcReqTpArray] -> MdRspOutDataSelc24/6(SrcReqTpArray)
  Constant23/1 -> MdRspOutDataSelc24/2(Index)
  [MdXXIsTargetPosAlready] -> MdRspOutDataSelc24/5(IsTargetPos32Bit_Val_read)
  [MdXX_QuitArray] -> MdRspOutDataSelc24/4(QuitArray)
  [modestate32] -> MdRspOutDataSelc24/1(modestate32_Val_read)
  MdRspOutDataSelc24/5(SrcReqTp) -> MdRsp24/5
  MdRspOutDataSelc24/4(IsTrgtPos) -> MdRsp24/4
  MdRspOutDataSelc24/3(Rsp) -> MdRsp24/3
  MdRspOutDataSelc25/3(Rsp) -> MdRsp25/3
  MdRspOutDataSelc25/4(IsTrgtPos) -> MdRsp25/4
  MdRspOutDataSelc25/5(SrcReqTp) -> MdRsp25/5
  [modestate32] -> MdRspOutDataSelc25/1(modestate32_Val_read)
  [MdXX_QuitArray] -> MdRspOutDataSelc25/4(QuitArray)
  [MdXXIsTargetPosAlready] -> MdRspOutDataSelc25/5(IsTargetPos32Bit_Val_read)
  Constant24/1 -> MdRspOutDataSelc25/2(Index)
  [MdXX_SrcReqTpArray] -> MdRspOutDataSelc25/6(SrcReqTpArray)
  [KeSMSuRspStatHldTm_Val] -> MdRspOutDataSelc25/3(KeSMSuRspStatHldTm_Val)
  MdRspOutDataSelc25/1(MdEn) -> MdRsp25/1
  MdRspOutDataSelc25/2(HldTm) -> MdRsp25/2
  MdRspOutDataSelc26/2(HldTm) -> MdRsp26/2
  MdRspOutDataSelc26/1(MdEn) -> MdRsp26/1
  [KeSMSuRspStatHldTm_Val] -> MdRspOutDataSelc26/3(KeSMSuRspStatHldTm_Val)
  [MdXX_SrcReqTpArray] -> MdRspOutDataSelc26/6(SrcReqTpArray)
  Constant25/1 -> MdRspOutDataSelc26/2(Index)
  [MdXXIsTargetPosAlready] -> MdRspOutDataSelc26/5(IsTargetPos32Bit_Val_read)
  [MdXX_QuitArray] -> MdRspOutDataSelc26/4(QuitArray)
  [modestate32] -> MdRspOutDataSelc26/1(modestate32_Val_read)
  MdRspOutDataSelc26/5(SrcReqTp) -> MdRsp26/5
  MdRspOutDataSelc26/4(IsTrgtPos) -> MdRsp26/4
  MdRspOutDataSelc26/3(Rsp) -> MdRsp26/3
  MdRspOutDataSelc27/3(Rsp) -> MdRsp27/3
  MdRspOutDataSelc27/4(IsTrgtPos) -> MdRsp27/4
  MdRspOutDataSelc27/5(SrcReqTp) -> MdRsp27/5
  [modestate32] -> MdRspOutDataSelc27/1(modestate32_Val_read)
  [MdXX_QuitArray] -> MdRspOutDataSelc27/4(QuitArray)
  [MdXXIsTargetPosAlready] -> MdRspOutDataSelc27/5(IsTargetPos32Bit_Val_read)
  Constant26/1 -> MdRspOutDataSelc27/2(Index)
  [MdXX_SrcReqTpArray] -> MdRspOutDataSelc27/6(SrcReqTpArray)
  [KeSMSuRspStatHldTm_Val] -> MdRspOutDataSelc27/3(KeSMSuRspStatHldTm_Val)
  MdRspOutDataSelc27/1(MdEn) -> MdRsp27/1
  MdRspOutDataSelc27/2(HldTm) -> MdRsp27/2
  MdRspOutDataSelc28/2(HldTm) -> MdRsp28/2
  MdRspOutDataSelc28/1(MdEn) -> MdRsp28/1
  [KeSMSuRspStatHldTm_Val] -> MdRspOutDataSelc28/3(KeSMSuRspStatHldTm_Val)
  [MdXX_SrcReqTpArray] -> MdRspOutDataSelc28/6(SrcReqTpArray)
  Constant27/1 -> MdRspOutDataSelc28/2(Index)
  [MdXXIsTargetPosAlready] -> MdRspOutDataSelc28/5(IsTargetPos32Bit_Val_read)
  [MdXX_QuitArray] -> MdRspOutDataSelc28/4(QuitArray)
  [modestate32] -> MdRspOutDataSelc28/1(modestate32_Val_read)
  MdRspOutDataSelc28/5(SrcReqTp) -> MdRsp28/5
  MdRspOutDataSelc28/4(IsTrgtPos) -> MdRsp28/4
  MdRspOutDataSelc28/3(Rsp) -> MdRsp28/3
  MdRspOutDataSelc29/3(Rsp) -> MdRsp29/3
  MdRspOutDataSelc29/4(IsTrgtPos) -> MdRsp29/4
  MdRspOutDataSelc29/5(SrcReqTp) -> MdRsp29/5
  [modestate32] -> MdRspOutDataSelc29/1(modestate32_Val_read)
  [MdXX_QuitArray] -> MdRspOutDataSelc29/4(QuitArray)
  [MdXXIsTargetPosAlready] -> MdRspOutDataSelc29/5(IsTargetPos32Bit_Val_read)
  Constant28/1 -> MdRspOutDataSelc29/2(Index)
  [MdXX_SrcReqTpArray] -> MdRspOutDataSelc29/6(SrcReqTpArray)
  [KeSMSuRspStatHldTm_Val] -> MdRspOutDataSelc29/3(KeSMSuRspStatHldTm_Val)
  MdRspOutDataSelc29/1(MdEn) -> MdRsp29/1
  MdRspOutDataSelc29/2(HldTm) -> MdRsp29/2
  MdRspOutDataSelc30/2(HldTm) -> MdRsp30/2
  MdRspOutDataSelc30/1(MdEn) -> MdRsp30/1
  [KeSMSuRspStatHldTm_Val] -> MdRspOutDataSelc30/3(KeSMSuRspStatHldTm_Val)
  [MdXX_SrcReqTpArray] -> MdRspOutDataSelc30/6(SrcReqTpArray)
  Constant29/1 -> MdRspOutDataSelc30/2(Index)
  [MdXXIsTargetPosAlready] -> MdRspOutDataSelc30/5(IsTargetPos32Bit_Val_read)
  [MdXX_QuitArray] -> MdRspOutDataSelc30/4(QuitArray)
  [modestate32] -> MdRspOutDataSelc30/1(modestate32_Val_read)
  MdRspOutDataSelc30/5(SrcReqTp) -> MdRsp30/5
  MdRspOutDataSelc30/4(IsTrgtPos) -> MdRsp30/4
  MdRspOutDataSelc30/3(Rsp) -> MdRsp30/3
  MdRspOutDataSelc31/3(Rsp) -> MdRsp31/3
  MdRspOutDataSelc31/4(IsTrgtPos) -> MdRsp31/4
  MdRspOutDataSelc31/5(SrcReqTp) -> MdRsp31/5
  [modestate32] -> MdRspOutDataSelc31/1(modestate32_Val_read)
  [MdXX_QuitArray] -> MdRspOutDataSelc31/4(QuitArray)
  [MdXXIsTargetPosAlready] -> MdRspOutDataSelc31/5(IsTargetPos32Bit_Val_read)
  Constant30/1 -> MdRspOutDataSelc31/2(Index)
  [MdXX_SrcReqTpArray] -> MdRspOutDataSelc31/6(SrcReqTpArray)
  [KeSMSuRspStatHldTm_Val] -> MdRspOutDataSelc31/3(KeSMSuRspStatHldTm_Val)
  MdRspOutDataSelc31/1(MdEn) -> MdRsp31/1
  MdRspOutDataSelc31/2(HldTm) -> MdRsp31/2
  MdRspOutDataSelc32/2(HldTm) -> MdRsp32/2
  MdRspOutDataSelc32/1(MdEn) -> MdRsp32/1
  [KeSMSuRspStatHldTm_Val] -> MdRspOutDataSelc32/3(KeSMSuRspStatHldTm_Val)
  [MdXX_SrcReqTpArray] -> MdRspOutDataSelc32/6(SrcReqTpArray)
  Constant31/1 -> MdRspOutDataSelc32/2(Index)
  [MdXXIsTargetPosAlready] -> MdRspOutDataSelc32/5(IsTargetPos32Bit_Val_read)
  [MdXX_QuitArray] -> MdRspOutDataSelc32/4(QuitArray)
  [modestate32] -> MdRspOutDataSelc32/1(modestate32_Val_read)
  MdRspOutDataSelc32/5(SrcReqTp) -> MdRsp32/5
  MdRspOutDataSelc32/4(IsTrgtPos) -> MdRsp32/4
  MdRspOutDataSelc32/3(Rsp) -> MdRsp32/3
  MdRsp21/1 -> Data Type Conversion21/1
  MdRsp22/1 -> Data Type Conversion22/1
  MdRsp23/1 -> Data Type Conversion23/1
  MdRsp24/1 -> Data Type Conversion24/1
  MdRsp25/1 -> Data Type Conversion25/1
  MdRsp26/1 -> Data Type Conversion26/1
  MdRsp27/1 -> Data Type Conversion27/1
  MdRsp28/1 -> Data Type Conversion28/1
  MdRsp29/1 -> Data Type Conversion29/1
  MdRsp30/1 -> Data Type Conversion30/1
  MdRsp31/1 -> Data Type Conversion31/1
  MdRsp32/1 -> Data Type Conversion32/1
  Data Type Conversion21/1 -> MdXX_RspOutComm_Md21_Rsp_write/1
  Data Type Conversion22/1 -> MdXX_RspOutComm_Md22_Rsp_write/1
  Data Type Conversion23/1 -> MdXX_RspOutComm_Md23_Rsp_write/1
  Data Type Conversion24/1 -> MdXX_RspOutComm_Md24_Rsp_write/1
  Data Type Conversion25/1 -> MdXX_RspOutComm_Md25_Rsp_write/1
  Data Type Conversion26/1 -> MdXX_RspOutComm_Md26_Rsp_write/1
  Data Type Conversion27/1 -> MdXX_RspOutComm_Md27_Rsp_write/1
  Data Type Conversion28/1 -> MdXX_RspOutComm_Md28_Rsp_write/1
  Data Type Conversion29/1 -> MdXX_RspOutComm_Md29_Rsp_write/1
  Data Type Conversion30/1 -> MdXX_RspOutComm_Md30_Rsp_write/1
  Data Type Conversion31/1 -> MdXX_RspOutComm_Md31_Rsp_write/1
  Data Type Conversion32/1 -> MdXX_RspOutComm_Md32_Rsp_write/1
  [LugAllEn] -> Switch/2
  Data Type Conversion8/1 -> Switch/3
  Switch/1 -> MdXX_RspOutComm_Md8_Rsp_write/1
  Constant32/1 -> Switch/1
  Data Type Conversion9/1 -> Switch1/3
  Constant33/1 -> Switch1/1
  [LugAllEn] -> Switch1/2
  Switch1/1 -> MdXX_RspOutComm_Md9_Rsp_write/1
  [VIPAllEn] -> Switch2/2
  Constant34/1 -> Switch2/1
  Data Type Conversion10/1 -> Switch2/3
  Switch2/1 -> MdXX_RspOutComm_Md10_Rsp_write/1
  Data Type Conversion12/1 -> Switch3/3
  Constant35/1 -> Switch3/1
  [VIPAllEn] -> Switch3/2
  Switch3/1 -> MdXX_RspOutComm_Md12_Rsp_write/1
  Constant36/1 -> Switch4/1
  Data Type Conversion14/1 -> Switch4/3
  [bed] -> Switch4/2
  MdRsp14/1 -> Data Type Conversion14/1
  Switch4/1 -> MdXX_RspOutComm_Md14_Rsp_write/1
  [bed] -> Switch5/2
  MdRsp15/1 -> Data Type Conversion15/1
  Data Type Conversion15/1 -> Switch5/3
  Constant37/1 -> Switch5/1

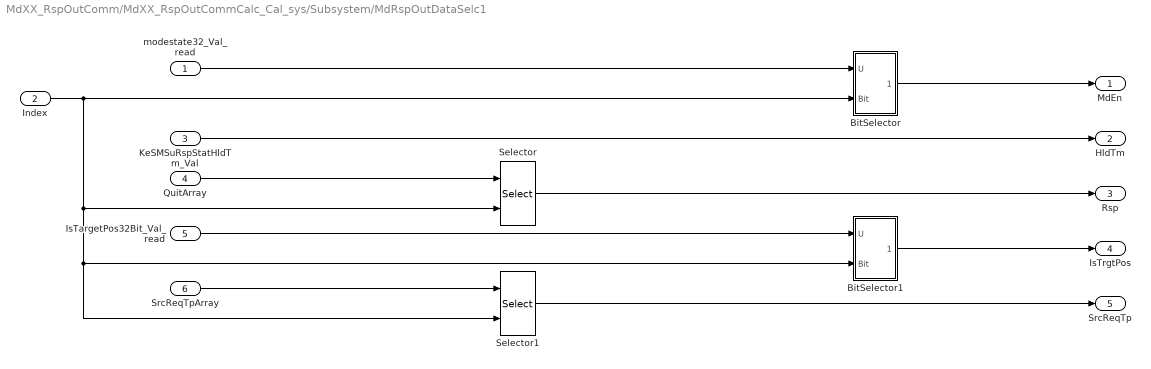
== system MdXX_RspOutComm/MdXX_RspOutCommCalc_Cal_sys/Subsystem/MdRspOutDataSelc1 ==
  modestate32_Val_read : Inport
  Index : Inport  Port=2
  KeSMSuRspStatHldTm_Val : Inport  Port=3
  QuitArray : Inport  Port=4
  IsTargetPos32Bit_Val_read : Inport  Port=5
  SrcReqTpArray : Inport  Port=6
  BitSelector : Subsystem
  BitSelector1 : Subsystem
  Selector : Selector  IndexMode=Zero-based  InputPortWidth=32  IndexOptions=Index vector (port)  Indices=[1 3]  OutputSizes=1
  Selector1 : Selector  IndexMode=Zero-based  InputPortWidth=32  IndexOptions=Index vector (port)  Indices=[1 3]  OutputSizes=1
  MdEn : Outport  VectorParamsAs1DForOutWhenUnconnected=off
  HldTm : Outport  Port=2  VectorParamsAs1DForOutWhenUnconnected=off
  Rsp : Outport  Port=3  VectorParamsAs1DForOutWhenUnconnected=off
  IsTrgtPos : Outport  Port=4  VectorParamsAs1DForOutWhenUnconnected=off
  SrcReqTp : Outport  Port=5  VectorParamsAs1DForOutWhenUnconnected=off
  wires:
  Selector1/1 -> SrcReqTp/1
  SrcReqTpArray/1 -> Selector1/1
  QuitArray/1 -> Selector/1
  IsTargetPos32Bit_Val_read/1 -> BitSelector1/1(U)
  BitSelector1/1(BitOut) -> IsTrgtPos/1
  modestate32_Val_read/1 -> BitSelector/1(U)
  BitSelector/1(BitOut) -> MdEn/1
  Selector/1 -> Rsp/1
  Index/1 -> BitSelector1/2(Bit), Selector1/2, Selector/2, BitSelector/2(Bit)
  KeSMSuRspStatHldTm_Val/1 -> HldTm/1

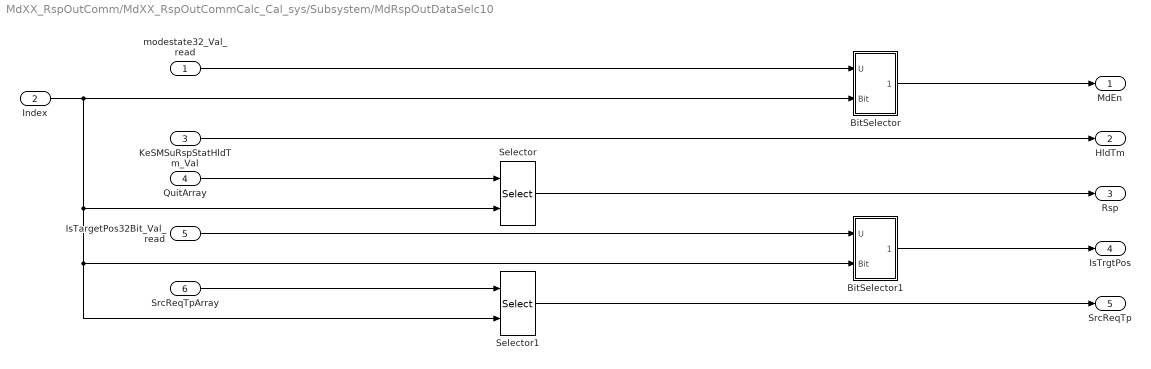
== system MdXX_RspOutComm/MdXX_RspOutCommCalc_Cal_sys/Subsystem/MdRspOutDataSelc10 ==
  modestate32_Val_read : Inport
  Index : Inport  Port=2
  KeSMSuRspStatHldTm_Val : Inport  Port=3
  QuitArray : Inport  Port=4
  IsTargetPos32Bit_Val_read : Inport  Port=5
  SrcReqTpArray : Inport  Port=6
  BitSelector : Subsystem
  BitSelector1 : Subsystem
  Selector : Selector  IndexMode=Zero-based  InputPortWidth=32  IndexOptions=Index vector (port)  Indices=[1 3]  OutputSizes=1
  Selector1 : Selector  IndexMode=Zero-based  InputPortWidth=32  IndexOptions=Index vector (port)  Indices=[1 3]  OutputSizes=1
  MdEn : Outport  VectorParamsAs1DForOutWhenUnconnected=off
  HldTm : Outport  Port=2  VectorParamsAs1DForOutWhenUnconnected=off
  Rsp : Outport  Port=3  VectorParamsAs1DForOutWhenUnconnected=off
  IsTrgtPos : Outport  Port=4  VectorParamsAs1DForOutWhenUnconnected=off
  SrcReqTp : Outport  Port=5  VectorParamsAs1DForOutWhenUnconnected=off
  wires:
  KeSMSuRspStatHldTm_Val/1 -> HldTm/1
  Index/1 -> BitSelector/2(Bit), Selector/2, Selector1/2, BitSelector1/2(Bit)
  Selector/1 -> Rsp/1
  BitSelector/1(BitOut) -> MdEn/1
  modestate32_Val_read/1 -> BitSelector/1(U)
  BitSelector1/1(BitOut) -> IsTrgtPos/1
  IsTargetPos32Bit_Val_read/1 -> BitSelector1/1(U)
  QuitArray/1 -> Selector/1
  SrcReqTpArray/1 -> Selector1/1
  Selector1/1 -> SrcReqTp/1

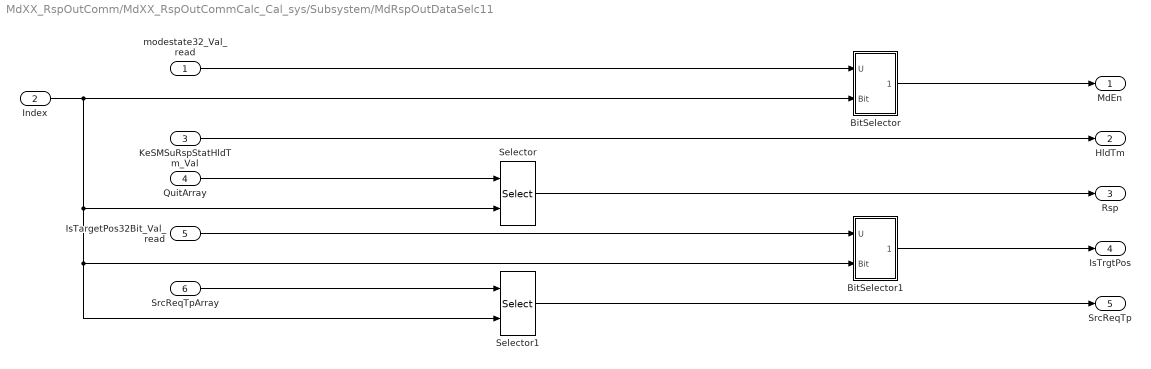
== system MdXX_RspOutComm/MdXX_RspOutCommCalc_Cal_sys/Subsystem/MdRspOutDataSelc11 ==
  modestate32_Val_read : Inport
  Index : Inport  Port=2
  KeSMSuRspStatHldTm_Val : Inport  Port=3
  QuitArray : Inport  Port=4
  IsTargetPos32Bit_Val_read : Inport  Port=5
  SrcReqTpArray : Inport  Port=6
  BitSelector : Subsystem
  BitSelector1 : Subsystem
  Selector : Selector  IndexMode=Zero-based  InputPortWidth=32  IndexOptions=Index vector (port)  Indices=[1 3]  OutputSizes=1
  Selector1 : Selector  IndexMode=Zero-based  InputPortWidth=32  IndexOptions=Index vector (port)  Indices=[1 3]  OutputSizes=1
  MdEn : Outport  VectorParamsAs1DForOutWhenUnconnected=off
  HldTm : Outport  Port=2  VectorParamsAs1DForOutWhenUnconnected=off
  Rsp : Outport  Port=3  VectorParamsAs1DForOutWhenUnconnected=off
  IsTrgtPos : Outport  Port=4  VectorParamsAs1DForOutWhenUnconnected=off
  SrcReqTp : Outport  Port=5  VectorParamsAs1DForOutWhenUnconnected=off
  wires:
  Selector1/1 -> SrcReqTp/1
  SrcReqTpArray/1 -> Selector1/1
  QuitArray/1 -> Selector/1
  IsTargetPos32Bit_Val_read/1 -> BitSelector1/1(U)
  BitSelector1/1(BitOut) -> IsTrgtPos/1
  modestate32_Val_read/1 -> BitSelector/1(U)
  BitSelector/1(BitOut) -> MdEn/1
  Selector/1 -> Rsp/1
  Index/1 -> BitSelector1/2(Bit), Selector1/2, Selector/2, BitSelector/2(Bit)
  KeSMSuRspStatHldTm_Val/1 -> HldTm/1

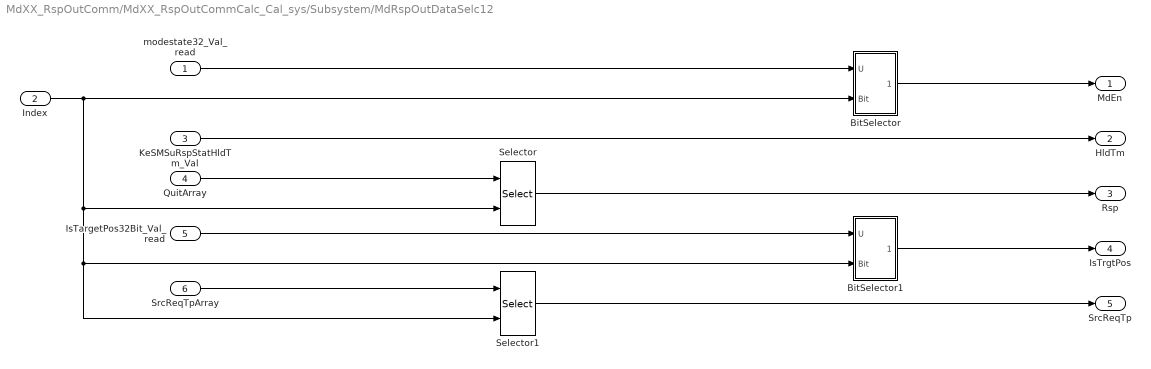
== system MdXX_RspOutComm/MdXX_RspOutCommCalc_Cal_sys/Subsystem/MdRspOutDataSelc12 ==
  modestate32_Val_read : Inport
  Index : Inport  Port=2
  KeSMSuRspStatHldTm_Val : Inport  Port=3
  QuitArray : Inport  Port=4
  IsTargetPos32Bit_Val_read : Inport  Port=5
  SrcReqTpArray : Inport  Port=6
  BitSelector : Subsystem
  BitSelector1 : Subsystem
  Selector : Selector  IndexMode=Zero-based  InputPortWidth=32  IndexOptions=Index vector (port)  Indices=[1 3]  OutputSizes=1
  Selector1 : Selector  IndexMode=Zero-based  InputPortWidth=32  IndexOptions=Index vector (port)  Indices=[1 3]  OutputSizes=1
  MdEn : Outport  VectorParamsAs1DForOutWhenUnconnected=off
  HldTm : Outport  Port=2  VectorParamsAs1DForOutWhenUnconnected=off
  Rsp : Outport  Port=3  VectorParamsAs1DForOutWhenUnconnected=off
  IsTrgtPos : Outport  Port=4  VectorParamsAs1DForOutWhenUnconnected=off
  SrcReqTp : Outport  Port=5  VectorParamsAs1DForOutWhenUnconnected=off
  wires:
  KeSMSuRspStatHldTm_Val/1 -> HldTm/1
  Index/1 -> BitSelector/2(Bit), Selector/2, Selector1/2, BitSelector1/2(Bit)
  Selector/1 -> Rsp/1
  BitSelector/1(BitOut) -> MdEn/1
  modestate32_Val_read/1 -> BitSelector/1(U)
  BitSelector1/1(BitOut) -> IsTrgtPos/1
  IsTargetPos32Bit_Val_read/1 -> BitSelector1/1(U)
  QuitArray/1 -> Selector/1
  SrcReqTpArray/1 -> Selector1/1
  Selector1/1 -> SrcReqTp/1

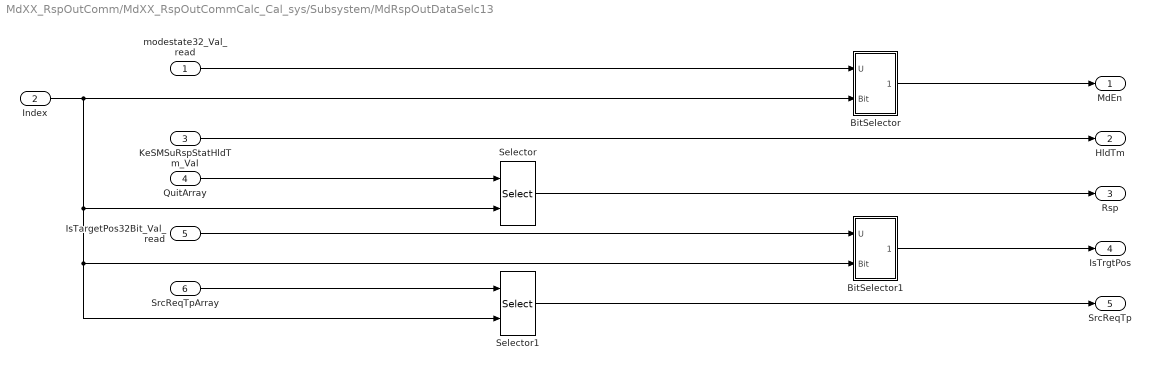
== system MdXX_RspOutComm/MdXX_RspOutCommCalc_Cal_sys/Subsystem/MdRspOutDataSelc13 ==
  modestate32_Val_read : Inport
  Index : Inport  Port=2
  KeSMSuRspStatHldTm_Val : Inport  Port=3
  QuitArray : Inport  Port=4
  IsTargetPos32Bit_Val_read : Inport  Port=5
  SrcReqTpArray : Inport  Port=6
  BitSelector : Subsystem
  BitSelector1 : Subsystem
  Selector : Selector  IndexMode=Zero-based  InputPortWidth=32  IndexOptions=Index vector (port)  Indices=[1 3]  OutputSizes=1
  Selector1 : Selector  IndexMode=Zero-based  InputPortWidth=32  IndexOptions=Index vector (port)  Indices=[1 3]  OutputSizes=1
  MdEn : Outport  VectorParamsAs1DForOutWhenUnconnected=off
  HldTm : Outport  Port=2  VectorParamsAs1DForOutWhenUnconnected=off
  Rsp : Outport  Port=3  VectorParamsAs1DForOutWhenUnconnected=off
  IsTrgtPos : Outport  Port=4  VectorParamsAs1DForOutWhenUnconnected=off
  SrcReqTp : Outport  Port=5  VectorParamsAs1DForOutWhenUnconnected=off
  wires:
  Selector1/1 -> SrcReqTp/1
  SrcReqTpArray/1 -> Selector1/1
  QuitArray/1 -> Selector/1
  IsTargetPos32Bit_Val_read/1 -> BitSelector1/1(U)
  BitSelector1/1(BitOut) -> IsTrgtPos/1
  modestate32_Val_read/1 -> BitSelector/1(U)
  BitSelector/1(BitOut) -> MdEn/1
  Selector/1 -> Rsp/1
  Index/1 -> BitSelector1/2(Bit), Selector1/2, Selector/2, BitSelector/2(Bit)
  KeSMSuRspStatHldTm_Val/1 -> HldTm/1

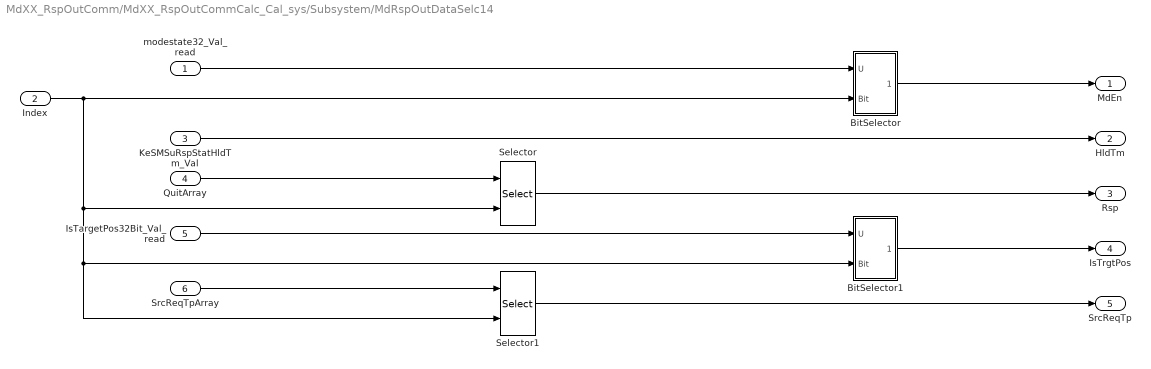
== system MdXX_RspOutComm/MdXX_RspOutCommCalc_Cal_sys/Subsystem/MdRspOutDataSelc14 ==
  modestate32_Val_read : Inport
  Index : Inport  Port=2
  KeSMSuRspStatHldTm_Val : Inport  Port=3
  QuitArray : Inport  Port=4
  IsTargetPos32Bit_Val_read : Inport  Port=5
  SrcReqTpArray : Inport  Port=6
  BitSelector : Subsystem
  BitSelector1 : Subsystem
  Selector : Selector  IndexMode=Zero-based  InputPortWidth=32  IndexOptions=Index vector (port)  Indices=[1 3]  OutputSizes=1
  Selector1 : Selector  IndexMode=Zero-based  InputPortWidth=32  IndexOptions=Index vector (port)  Indices=[1 3]  OutputSizes=1
  MdEn : Outport  VectorParamsAs1DForOutWhenUnconnected=off
  HldTm : Outport  Port=2  VectorParamsAs1DForOutWhenUnconnected=off
  Rsp : Outport  Port=3  VectorParamsAs1DForOutWhenUnconnected=off
  IsTrgtPos : Outport  Port=4  VectorParamsAs1DForOutWhenUnconnected=off
  SrcReqTp : Outport  Port=5  VectorParamsAs1DForOutWhenUnconnected=off
  wires:
  KeSMSuRspStatHldTm_Val/1 -> HldTm/1
  Index/1 -> BitSelector/2(Bit), Selector/2, Selector1/2, BitSelector1/2(Bit)
  Selector/1 -> Rsp/1
  BitSelector/1(BitOut) -> MdEn/1
  modestate32_Val_read/1 -> BitSelector/1(U)
  BitSelector1/1(BitOut) -> IsTrgtPos/1
  IsTargetPos32Bit_Val_read/1 -> BitSelector1/1(U)
  QuitArray/1 -> Selector/1
  SrcReqTpArray/1 -> Selector1/1
  Selector1/1 -> SrcReqTp/1

== system MdXX_RspOutComm/MdXX_RspOutCommCalc_Cal_sys/Subsystem/MdRspOutDataSelc15 ==
  modestate32_Val_read : Inport
  Index : Inport  Port=2
  KeSMSuRspStatHldTm_Val : Inport  Port=3
  QuitArray : Inport  Port=4
  IsTargetPos32Bit_Val_read : Inport  Port=5
  SrcReqTpArray : Inport  Port=6
  BitSelector : Subsystem
  BitSelector1 : Subsystem
  Selector : Selector  IndexMode=Zero-based  InputPortWidth=32  IndexOptions=Index vector (port)  Indices=[1 3]  OutputSizes=1
  Selector1 : Selector  IndexMode=Zero-based  InputPortWidth=32  IndexOptions=Index vector (port)  Indices=[1 3]  OutputSizes=1
  MdEn : Outport  VectorParamsAs1DForOutWhenUnconnected=off
  HldTm : Outport  Port=2  VectorParamsAs1DForOutWhenUnconnected=off
  Rsp : Outport  Port=3  VectorParamsAs1DForOutWhenUnconnected=off
  IsTrgtPos : Outport  Port=4  VectorParamsAs1DForOutWhenUnconnected=off
  SrcReqTp : Outport  Port=5  VectorParamsAs1DForOutWhenUnconnected=off
  wires:
  Selector1/1 -> SrcReqTp/1
  SrcReqTpArray/1 -> Selector1/1
  QuitArray/1 -> Selector/1
  IsTargetPos32Bit_Val_read/1 -> BitSelector1/1(U)
  BitSelector1/1(BitOut) -> IsTrgtPos/1
  modestate32_Val_read/1 -> BitSelector/1(U)
  BitSelector/1(BitOut) -> MdEn/1
  Selector/1 -> Rsp/1
  Index/1 -> BitSelector1/2(Bit), Selector1/2, Selector/2, BitSelector/2(Bit)
  KeSMSuRspStatHldTm_Val/1 -> HldTm/1
